simulink model "HVDCThyristorBased"  (R2024b)
settings: Solver=FixedStepDiscrete  StartTime=0.0  StopTime=2  FixedStep=Ts  RelTol=1e-3  AbsTol=1e-2
InitFcn:
  | Ts=50e-6;
  | 
  | % Rectifier AC side :
  | VLL_nom_R = 500e3; % V
  | Fnom_R = 60;           % Hz
  | 
  | % Inverter AC side :
  | VLL_nom_I = 345e3; % V
  | Fnom_I = 50;           % Hz
  | 
  | % DC :
  | Vdc_nom = 500e3;   % V
  | Idc_nom  = 2000;     % A
undefined symbols (not defined in the file or in its folder): D1, Delta, lagging, pulse, test_alpha
libraries: simulink x24, spsOnDelayLib x12, spsFirstOrderFilterLib x9, spsSampleandHoldLib x8, spsMultimeterLib x7, spsMonostableLib x7, spsThreePhaseHarmonicFilterLib x6, spsEdgeDetectorLib x6, spsGroundLib x4, spsUniversalBridgeLib x4, spsImpedanceMeasurementLib x3, spsBistableLib x3
(part 3 of 5)

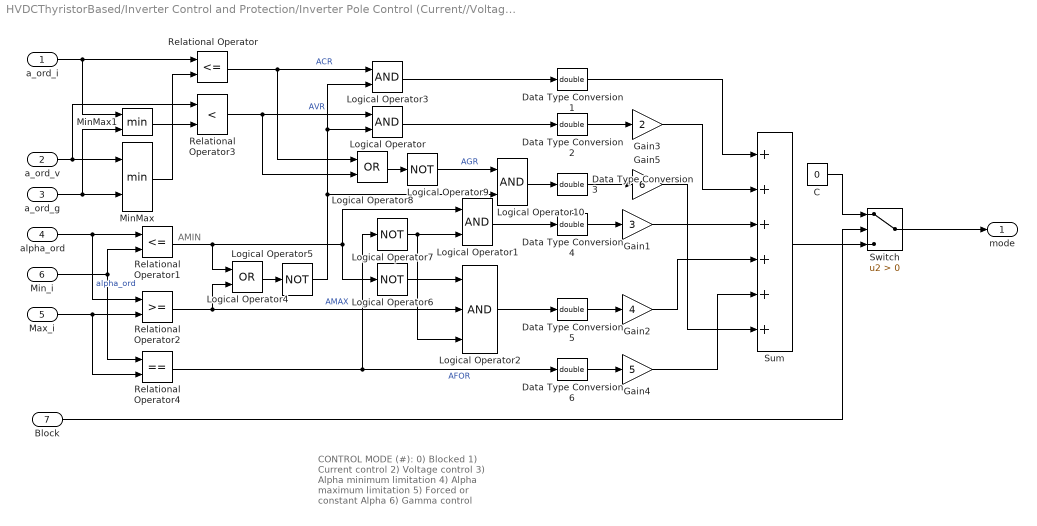
== system HVDCThyristorBased/Inverter Control and Protection/Inverter Pole Control (Current//Voltage//Gamma)/Control Mode  ==
  note: AMIN
  note: CONTROL MODE (#):
      |
      | 0) Blocked
      | 1) Current control
      | 2) Voltage control
      | 3) Alpha minimum limitation
      | 4) Alpha maximum limitation
      | 5) Forced or constant Alpha
      | 6) Gamma control
  "a_ord_i " : Inport
  a_ord_v : Inport  Port=2
  a_ord_g : Inport  Port=3
  alpha_ord : Inport  Port=4
  Max_i : Inport  Port=5
  Min_i : Inport  Port=6
  Block : Inport  Port=7
  C : Constant  Value=0
  Data Type Conversion{1..6} (6 alike) : DataTypeConversion  OutDataTypeStr=double  SaturateOnIntegerOverflow=off  RndMeth=Floor
  Gain1 : Gain  Gain=3  OutDataTypeStr=double  SaturateOnIntegerOverflow=on  ParamDataTypeStr=Inherit: Same as input
  Gain2 : Gain  Gain=4  OutDataTypeStr=double  SaturateOnIntegerOverflow=on  ParamDataTypeStr=Inherit: Same as input
  Gain3 : Gain  Gain=2  OutDataTypeStr=double  SaturateOnIntegerOverflow=on  ParamDataTypeStr=Inherit: Same as input
  Gain4 : Gain  Gain=5  OutDataTypeStr=double  SaturateOnIntegerOverflow=on  ParamDataTypeStr=Inherit: Same as input
  Gain5 : Gain  Gain=6  OutDataTypeStr=double  SaturateOnIntegerOverflow=on  ParamDataTypeStr=Inherit: Same as input
  Logical Operator{,1,3,10} (4 alike) : Logic
  Logical Operator2 : Logic  Inputs=3
  Logical Operator4 : Logic  Operator=OR
  Logical Operator{5..7,9} (4 alike) : Logic  Operator=NOT
  Logical Operator8 : Logic  Operator=OR
  MinMax : MinMax  Inputs=2  InputSameDT=on  SaturateOnIntegerOverflow=on
  MinMax1 : MinMax  Inputs=2  InputSameDT=on  SaturateOnIntegerOverflow=on
  Relational Operator : RelationalOperator  Operator=<=
  Relational Operator1 : RelationalOperator  Operator=<=
  Relational Operator2 : RelationalOperator
  Relational Operator3 : RelationalOperator  Operator=<
  Relational Operator4 : RelationalOperator  Operator===
  Sum : Sum  Inputs=++++++  InputSameDT=on  SaturateOnIntegerOverflow=on  OutDataTypeStr=Inherit: Same as first input
  Switch : Switch  Criteria=u2 > Threshold
  mode : Outport  VectorParamsAs1DForOutWhenUnconnected=off
  wires:
  Data Type Conversion6/1 -> Gain4/1
  Data Type Conversion5/1 -> Gain2/1
  Data Type Conversion4/1 -> Gain1/1
  Data Type Conversion3/1 -> Gain5/1
  Data Type Conversion2/1 -> Gain3/1
  Data Type Conversion1/1 -> Sum/1
  Switch/1 -> mode/1
  Logical Operator5/1 -> Logical Operator3/2, Logical Operator/2, Logical Operator10/2
  Logical Operator7/1 -> Logical Operator2/3, Logical Operator1/2
  Gain4/1 -> Sum/5
  Logical Operator1/1 -> Data Type Conversion4/1
  Relational Operator4/1 -> Logical Operator7/1, Data Type Conversion6/1  "AFOR"
  Max_i/1 -> Relational Operator4/2, Relational Operator2/2
  Min_i/1 -> Relational Operator4/1, Relational Operator1/2
  Gain2/1 -> Sum/4
  Gain1/1 -> Sum/3
  Logical Operator2/1 -> Data Type Conversion5/1
  Logical Operator6/1 -> Logical Operator2/1
  Relational Operator2/1 -> Logical Operator2/2, Logical Operator4/2  "AMAX"
  Logical Operator4/1 -> Logical Operator5/1
  Relational Operator1/1 -> Logical Operator1/1, Logical Operator6/1, Logical Operator4/1
  alpha_ord/1 -> Relational Operator2/1, Relational Operator1/1  "alpha_ord"
  Logical Operator/1 -> Data Type Conversion2/1
  Relational Operator3/1 -> Logical Operator/1, Logical Operator8/2  "AVR"
  Gain3/1 -> Sum/2
  Logical Operator3/1 -> Data Type Conversion1/1
  Relational Operator/1 -> Logical Operator3/1, Logical Operator8/1  "ACR"
  "a_ord_i "/1 -> Relational Operator/1, MinMax1/1
  Block/1 -> Switch/2
  Sum/1 -> Switch/3
  C/1 -> Switch/1
  a_ord_v/1 -> MinMax/1, Relational Operator3/1
  a_ord_g/1 -> MinMax/2, MinMax1/2
  MinMax/1 -> Relational Operator/2
  Logical Operator8/1 -> Logical Operator9/1
  Gain5/1 -> Sum/6
  MinMax1/1 -> Relational Operator3/2
  Logical Operator9/1 -> Logical Operator10/1  "AGR"
  Logical Operator10/1 -> Data Type Conversion3/1

== system HVDCThyristorBased/Inverter Control and Protection/Inverter Pole Control (Current//Voltage//Gamma)/Current Regulator ==
  note: Current Regulator
  Max_i : Inport
  Min_i : Inport  Port=2
  ERR : Inport  Port=3
  Max_pi : Inport  Port=4
  Min_pi : Inport  Port=5
  Alpha_lin : Inport  Port=6
  Max_lin : Inport  Port=7
  Min_lin : Inport  Port=8
  Inv : Inport  Port=9
  PI Regulator with external limits and linrarized Kp (Discrete) : Subsystem  mask(PI Regulator  With  External  Limits (Discrete)){Kp=Kp_I, Ki=Ki_I, IC_i=ICi_I, On_lin=on, pas=Ts}
      mask prompts: Kp "Kp (deg/pu):"; Ki "Ki (deg/pu/s):"; IC_i "Integrator Initial Condition (deg):"; On_lin "Linearization  (On)"; pas "Sample time (s):"
      mask help: For the linearization it is important to specifie the mode of operation i.e. rectifier or inverter (negation of rectifier).
      mask Display: disp('PI Regulator\nWith external limits\n(Linearized Kp)\n(Discrete)\n\n')
  Alpha_ord : Outport  VectorParamsAs1DForOutWhenUnconnected=off
  wires:
  PI Regulator with external limits and linrarized Kp (Discrete)/1(Alpha_ord) -> Alpha_ord/1
  Max_i/1 -> PI Regulator with external limits and linrarized Kp (Discrete)/1(Max_i)
  Min_i/1 -> PI Regulator with external limits and linrarized Kp (Discrete)/2(Min_i)
  ERR/1 -> PI Regulator with external limits and linrarized Kp (Discrete)/3(ERR)
  Max_pi/1 -> PI Regulator with external limits and linrarized Kp (Discrete)/4(Max_pi)
  Min_pi/1 -> PI Regulator with external limits and linrarized Kp (Discrete)/5(Min_pi)
  Alpha_lin/1 -> PI Regulator with external limits and linrarized Kp (Discrete)/6(Alpha_lin)
  Max_lin/1 -> PI Regulator with external limits and linrarized Kp (Discrete)/7(Max_lin)
  Min_lin/1 -> PI Regulator with external limits and linrarized Kp (Discrete)/8(Min_lin)
  Inv/1 -> PI Regulator with external limits and linrarized Kp (Discrete)/9(Inv)

== system HVDCThyristorBased/Inverter Control and Protection/Inverter Pole Control (Current//Voltage//Gamma)/Gamma Error ==
  note: Gamma Error
  G_ref : Inport
  G_meas : Inport  Port=2
  Block : Inport  Port=3
  Id_err : Inport  Port=4
  Enable (Held) : EnablePort  PropagateVarSize=During execution
  Constant1 : Constant  Value=0
  Constant2 : Constant  Value=0
  Constant3 : Constant  Value=G_marg
  Constant4 : Constant  Value=Id_marg
  First-Order Filter (T=0.01) : spsFirstOrderFilterLib/First-Order Filter  FilterType=Lowpass  Tc=0.01  Ts=Ts  Initialize=off  Vac_Init=[0, 0, 60]  Vdc_Init=0  PlotResponse=off  FreqRange="[0,  200,  1]"
  MIN:eps MAX:inf : Saturate  UpperLimit=inf  LowerLimit=eps
  Math Function : Math  Operator=reciprocal  SignedPower=on
  Product1 : Product  Inputs=3  InputSameDT=on  SaturateOnIntegerOverflow=on  OutDataTypeStr=Inherit: Same as first input
  Saturation Dynamic : simulink/Discontinuities/Saturation Dynamic  OutMin=[]  OutMax=[]  OutDataTypeStr=Inherit: Same as second input  OutDataType=fixdt(1, 16)  OutScaling=2^-10  DoSatur=off
  Sum3 : Sum  Inputs=-+-  InputSameDT=on  SaturateOnIntegerOverflow=on  OutDataTypeStr=Inherit: Same as first input
  Switch2 : Switch  Criteria=u2 > Threshold
  ERR_G : Outport  VectorParamsAs1DForOutWhenUnconnected=off
  wires:
  Saturation Dynamic/1 -> Product1/3
  Sum3/1 -> Switch2/3
  G_ref/1 -> Sum3/1
  G_meas/1 -> Sum3/2
  Constant1/1 -> Switch2/1
  Block/1 -> Switch2/2
  Switch2/1 -> ERR_G/1  "ERR"
  Constant2/1 -> Saturation Dynamic/3
  Math Function/1 -> Product1/2
  MIN:eps MAX:inf/1 -> Math Function/1
  Constant4/1 -> MIN:eps MAX:inf/1, Saturation Dynamic/1
  Product1/1 -> First-Order Filter (T=0.01)/1
  First-Order Filter (T=0.01)/1 -> Sum3/3  "dG"
  Id_err/1 -> Saturation Dynamic/2
  Constant3/1 -> Product1/1

== system HVDCThyristorBased/Inverter Control and Protection/Inverter Pole Control (Current//Voltage//Gamma)/Gamma Regulator ==
  note: Gamma Regulator
  Max_i : Inport
  Min_i : Inport  Port=2
  ERR : Inport  Port=3
  Max_pi : Inport  Port=4
  Min_pi : Inport  Port=5
  Alpha_lin : Inport  Port=6
  Max_lin : Inport  Port=7
  Min_lin : Inport  Port=8
  Inv : Inport  Port=9
  Enable (Held) : EnablePort  PropagateVarSize=During execution
  PI Regulator with external limits and linrarized Kp (Discrete)1 : Subsystem  mask(PI Regulator  With  External  Limits (Discrete)){Kp=Kp_G, Ki=Ki_G, IC_i=ICi_G, On_lin=on, pas=Ts}
      mask prompts: Kp "Kp (deg/pu):"; Ki "Ki (deg/pu/s):"; IC_i "Integrator Initial Condition (deg):"; On_lin "Linearization  (On)"; pas "Sample time (s):"
      mask help: For the linearization it is important to specifie the mode of operation i.e. rectifier or inverter (negation of rectifier).
      mask Display: disp('PI Regulator\nWith external limits\n(Linearized Kp)\n(Discrete)\n\n')
  Alpha_ord : Outport  VectorParamsAs1DForOutWhenUnconnected=off
  wires:
  PI Regulator with external limits and linrarized Kp (Discrete)1/1(Alpha_ord) -> Alpha_ord/1
  Max_i/1 -> PI Regulator with external limits and linrarized Kp (Discrete)1/1(Max_i)
  Min_i/1 -> PI Regulator with external limits and linrarized Kp (Discrete)1/2(Min_i)
  ERR/1 -> PI Regulator with external limits and linrarized Kp (Discrete)1/3(ERR)
  Max_pi/1 -> PI Regulator with external limits and linrarized Kp (Discrete)1/4(Max_pi)
  Min_pi/1 -> PI Regulator with external limits and linrarized Kp (Discrete)1/5(Min_pi)
  Alpha_lin/1 -> PI Regulator with external limits and linrarized Kp (Discrete)1/6(Alpha_lin)
  Max_lin/1 -> PI Regulator with external limits and linrarized Kp (Discrete)1/7(Max_lin)
  Min_lin/1 -> PI Regulator with external limits and linrarized Kp (Discrete)1/8(Min_lin)
  Inv/1 -> PI Regulator with external limits and linrarized Kp (Discrete)1/9(Inv)

== system HVDCThyristorBased/Inverter Control and Protection/Inverter Pole Control (Current//Voltage//Gamma)/Voltage Error ==
  note: Voltage Error
  Vd_ref : Inport
  Vd_meas : Inport  Port=2
  Block : Inport  Port=3
  Id_err : Inport  Port=4
  Enable (Held) : EnablePort  PropagateVarSize=During execution
  Constant1 : Constant  Value=0
  Constant2 : Constant  Value=0
  Constant3 : Constant  Value=Vd_marg
  Constant4 : Constant  Value=Id_marg
  First-Order Filter (T = 0.1) : spsFirstOrderFilterLib/First-Order Filter  FilterType=Lowpass  Tc=0.01  Ts=Ts  Initialize=on  Vac_Init=[0, 0, 60]  Vdc_Init=0  PlotResponse=off  FreqRange="[0,  200,  1]"
  MIN:eps MAX:inf : Saturate  UpperLimit=inf  LowerLimit=eps
  Math Function : Math  Operator=reciprocal  SignedPower=on
  Product1 : Product  Inputs=3  InputSameDT=on  SaturateOnIntegerOverflow=on  OutDataTypeStr=Inherit: Same as first input
  Saturation Dynamic : simulink/Discontinuities/Saturation Dynamic  OutMin=[]  OutMax=[]  OutDataTypeStr=Inherit: Same as second input  OutDataType=fixdt(1, 16)  OutScaling=2^-10  DoSatur=off
  Sum3 : Sum  Inputs=+--  InputSameDT=on  SaturateOnIntegerOverflow=on  OutDataTypeStr=Inherit: Same as first input
  Switch2 : Switch  Criteria=u2 > Threshold
  ERR_V : Outport  VectorParamsAs1DForOutWhenUnconnected=off
  wires:
  Saturation Dynamic/1 -> Product1/3
  Constant3/1 -> Product1/1
  Id_err/1 -> Saturation Dynamic/2
  First-Order Filter (T = 0.1)/1 -> Sum3/3  "dV"
  Product1/1 -> First-Order Filter (T = 0.1)/1
  Constant4/1 -> MIN:eps MAX:inf/1, Saturation Dynamic/1
  MIN:eps MAX:inf/1 -> Math Function/1
  Math Function/1 -> Product1/2
  Constant2/1 -> Saturation Dynamic/3
  Switch2/1 -> ERR_V/1  "ERR"
  Block/1 -> Switch2/2
  Constant1/1 -> Switch2/1
  Vd_meas/1 -> Sum3/2
  Vd_ref/1 -> Sum3/1
  Sum3/1 -> Switch2/3

== system HVDCThyristorBased/Inverter Control and Protection/Inverter Pole Control (Current//Voltage//Gamma)/Voltage Regulator ==
  note: Voltage Regulator
  Max_i : Inport
  Min_i : Inport  Port=2
  ERR : Inport  Port=3
  Max_pi : Inport  Port=4
  Min_pi : Inport  Port=5
  Alpha_lin : Inport  Port=6
  Max_lin : Inport  Port=7
  Min_lin : Inport  Port=8
  Inv : Inport  Port=9
  Enable (Held) : EnablePort  PropagateVarSize=During execution
  PI Regulator with external limits and linrarized Kp (Discrete) : Subsystem  mask(PI Regulator  With  External  Limits (Discrete)){Kp=Kp_V, Ki=Ki_V, IC_i=ICi_V, On_lin=on, pas=Ts}
      mask prompts: Kp "Kp (deg/pu):"; Ki "Ki (deg/pu/s):"; IC_i "Integrator Initial Condition (deg):"; On_lin "Linearization  (On)"; pas "Sample time (s):"
      mask help: For the linearization it is important to specifie the mode of operation i.e. rectifier or inverter (negation of rectifier).
      mask Display: disp('PI Regulator\nWith external limits\n(Linearized Kp)\n(Discrete)\n\n')
  Alpha_ord : Outport  VectorParamsAs1DForOutWhenUnconnected=off
  wires:
  Inv/1 -> PI Regulator with external limits and linrarized Kp (Discrete)/9(Inv)
  Min_lin/1 -> PI Regulator with external limits and linrarized Kp (Discrete)/8(Min_lin)
  Max_lin/1 -> PI Regulator with external limits and linrarized Kp (Discrete)/7(Max_lin)
  Alpha_lin/1 -> PI Regulator with external limits and linrarized Kp (Discrete)/6(Alpha_lin)
  Min_pi/1 -> PI Regulator with external limits and linrarized Kp (Discrete)/5(Min_pi)
  Max_pi/1 -> PI Regulator with external limits and linrarized Kp (Discrete)/4(Max_pi)
  ERR/1 -> PI Regulator with external limits and linrarized Kp (Discrete)/3(ERR)
  Min_i/1 -> PI Regulator with external limits and linrarized Kp (Discrete)/2(Min_i)
  Max_i/1 -> PI Regulator with external limits and linrarized Kp (Discrete)/1(Max_i)
  PI Regulator with external limits and linrarized Kp (Discrete)/1(Alpha_ord) -> Alpha_ord/1

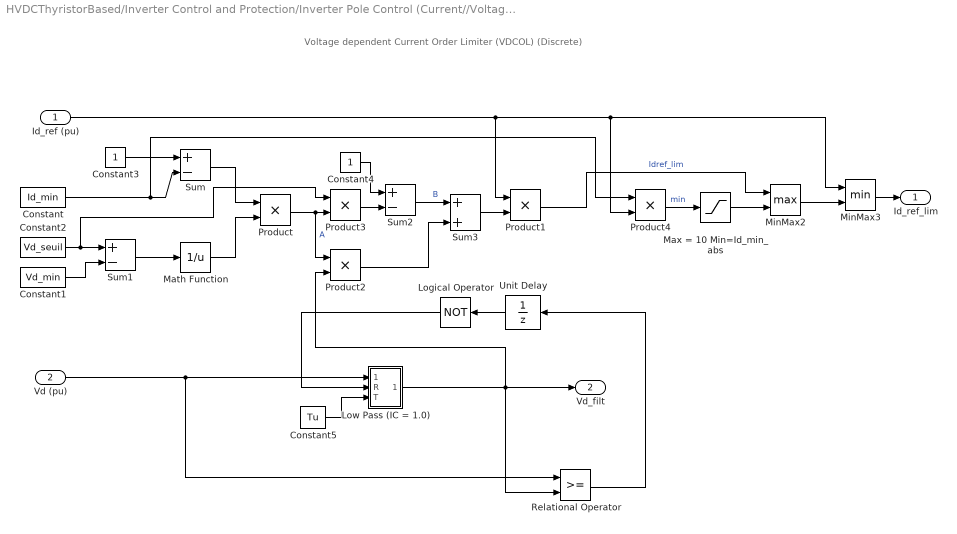
== system HVDCThyristorBased/Inverter Control and Protection/Inverter Pole Control (Current//Voltage//Gamma)/Voltage dependent Current Order Limiter ==
  note: Voltage dependent Current Order Limiter (VDCOL) (Discrete)
  Id_ref (pu) : Inport
  Vd (pu) : Inport  Port=2
  Constant : Constant  Value=Id_min
  Constant1 : Constant  Value=Vd_min
  Constant2 : Constant  Value=Vd_seuil
  Constant3 : Constant
  Constant4 : Constant
  Constant5 : Constant  Value=Tu
  Logical Operator : Logic  Operator=NOT
  Low Pass (IC = 1.0) : Subsystem  mask(Low Pass Filter With Reset (discrete: Zoh method, Forward Euler)){ic=1, dt=Ts}
      mask prompts: ic "Initial condition:"; dt "Sample time (s)"
      mask help:
      | The output will be reset to the input value (Time constant = 0)  during the input (2) is True. The Time constant (T) is defined by
      | input (3).
      mask Display:
      | plot(0,0,100,100,[90,80,70,60,50,40,29,20,10],[60,55,52,55,60,65,67,65,60],[89,80,71,60,50,40,30,20,10],[40,35,32,35,40,45,47,45,40],[56,44],[70,50]);
      | disp('\n\nD')
  Math Function : Math  Operator=reciprocal  SignedPower=on
  Max = 10 Min=Id_min_abs : Saturate  UpperLimit=10  LowerLimit=Id_min_abs
  MinMax2 : MinMax  Function=max  Inputs=2  InputSameDT=on  SaturateOnIntegerOverflow=on
  MinMax3 : MinMax  Inputs=2  InputSameDT=on  SaturateOnIntegerOverflow=on
  Product{,1..4} (5 alike) : Product  InputSameDT=on  SaturateOnIntegerOverflow=on  OutDataTypeStr=Inherit: Same as first input
  Relational Operator : RelationalOperator
  Sum : Sum  Inputs=+-  InputSameDT=on  SaturateOnIntegerOverflow=on  OutDataTypeStr=Inherit: Same as first input
  Sum1 : Sum  Inputs=+-  InputSameDT=on  SaturateOnIntegerOverflow=on  OutDataTypeStr=Inherit: Same as first input
  Sum2 : Sum  Inputs=+-  InputSameDT=on  SaturateOnIntegerOverflow=on  OutDataTypeStr=Inherit: Same as first input
  Sum3 : Sum  InputSameDT=on  SaturateOnIntegerOverflow=on  OutDataTypeStr=Inherit: Same as first input
  Unit Delay : UnitDelay  SampleTime=Ts  HasFrameUpgradeWarning=on
  Id_ref_lim : Outport  InitialOutput=0  VectorParamsAs1DForOutWhenUnconnected=off
  Vd_filt : Outport  Port=2  InitialOutput=0  VectorParamsAs1DForOutWhenUnconnected=off
  wires:
  Relational Operator/1 -> Unit Delay/1
  Max = 10 Min=Id_min_abs/1 -> MinMax2/2
  MinMax2/1 -> MinMax3/2
  Product1/1 -> MinMax2/1  "Idref_lim"
  Constant2/1 -> Product3/1, Sum1/1
  Product/1 -> Product3/2, Product2/1  "A"
  Product3/1 -> Sum2/2
  MinMax3/1 -> Id_ref_lim/1
  Id_ref (pu)/1 -> Product4/2, MinMax3/1, Product1/1
  Product4/1 -> Max = 10 Min=Id_min_abs/1  "min"
  Constant/1 -> Product4/1, Sum/2
  Sum3/1 -> Product1/2
  Product2/1 -> Sum3/2
  Sum2/1 -> Sum3/1  "B"
  Constant4/1 -> Sum2/1
  Math Function/1 -> Product/2
  Sum/1 -> Product/1
  Sum1/1 -> Math Function/1
  Constant1/1 -> Sum1/2
  Constant3/1 -> Sum/1
  Constant5/1 -> Low Pass (IC = 1.0)/3(T)
  Low Pass (IC = 1.0)/1(Out) -> Vd_filt/1, Relational Operator/2, Product2/2
  Vd (pu)/1 -> Relational Operator/1, Low Pass (IC = 1.0)/1(In)
  Unit Delay/1 -> Logical Operator/1
  Logical Operator/1 -> Low Pass (IC = 1.0)/2(R)

== system HVDCThyristorBased/Inverter Control and Protection/Inverter Pole Control (Current//Voltage//Gamma)/alpha_init ==
  In1 : Inport  PortDimensions=1
  IC : InitialCondition  Value=min([ICi_V,ICi_I,ICi_G])
  Out1 : Outport  VectorParamsAs1DForOutWhenUnconnected=off
  wires:
  IC/1 -> Out1/1
  In1/1 -> IC/1

== system HVDCThyristorBased/Inverter Control and Protection/Inverter Protections/Commutation Failure Prevention Control (CFPREV) ==
  note: Commutation failure Prevention Control Module (CFPREV)
  Uabc (pu) : Inport
  C : Constant  Value=STATE
  CFPREV : Subsystem  TreatAsAtomicUnit=on
  AMIN_CFPREV (deg) : Outport  VectorParamsAs1DForOutWhenUnconnected=off
  wires:
  C/1 -> CFPREV/Enable
  Uabc (pu)/1 -> CFPREV/1(Uabc (pu))
  CFPREV/1(AMIN_CFPREV (deg)) -> AMIN_CFPREV (deg)/1

== system HVDCThyristorBased/Inverter Control and Protection/Inverter Protections/Informations ==
  note: The CFPREV  mitigates commutation failures due to AC voltage dips. After a fault detection (three-phase or
      | one-phase) an angle value (AMIN_CFPREV) is sent to the converter control in order to be deducted from the
      | maximum delay angle limit (alpha_max). In practice, the commutation margin is consequently enlarged
      | reducing therefore the risk of commutation failures (note 1).
  note: The Commutation failure prevention control (CFPREV) and the Low AC voltage detection (LACVD)
      | constitutes the protective functions at the rinverter.
  note: The LACVD detects a low AC voltage condition on the inverter commutation bus and sends a signal
      | (Lock) to the DCPROT (in the rectifier) in order to prevent the detection of a DC fault when the drop in
      | the DC voltage is due to a fault on the AC side. The LACVD at the irectifier sends also a signal to
      | lock the DCPROT for the same reason.
  note: DESCRIPTION
  note: DC Protections - Inverter
  note: NOTE 1: Result of a failure of the incoming valve to take over the direct current before the commutating voltage reverses its polarity.

== system HVDCThyristorBased/Inverter Control and Protection/Inverter Protections/Low  AC Voltage Detection (LACVD) ==
  note: Low AC Voltage Detection
  Uac (pu) : Inport
  Enable (Held) : EnablePort  PropagateVarSize=During execution  ShowOutputPort=on
  C : Constant  Value=STATE
  LACVD : Subsystem  TreatAsAtomicUnit=on
  Logical Operator : Logic  AllPortsSameDT=off
  Low_AC_Voltage : Outport  VectorParamsAs1DForOutWhenUnconnected=off
  wires:
  Uac (pu)/1 -> LACVD/1(Uac (pu))
  LACVD/1(Low_AC_Voltage) -> Low_AC_Voltage/1
  Enable (Held)/1 -> Logical Operator/1
  Logical Operator/1 -> LACVD/Enable
  C/1 -> Logical Operator/2

== system HVDCThyristorBased/Inverter Control and Protection/Inverter Protections/Udio_6p ==
  note: Three-phase full-wave rectification
  Uabc (pu) : Inport
  MinMax : MinMax  Function=max  InputSameDT=on  SaturateOnIntegerOverflow=on
  MinMax1 : MinMax  InputSameDT=on  SaturateOnIntegerOverflow=on
  Sum : Sum  Inputs=+-  InputSameDT=on  SaturateOnIntegerOverflow=on  OutDataTypeStr=Inherit: Same as first input
  conversion pu ac->dc : Gain  Gain=pi/(3*sqrt(3))  SaturateOnIntegerOverflow=on  OutDataTypeStr=Inherit: Same as input  ParamDataTypeStr=Inherit: Same as input
  Udio_6p : Outport  VectorParamsAs1DForOutWhenUnconnected=off
  wires:
  conversion pu ac->dc/1 -> Udio_6p/1
  Sum/1 -> conversion pu ac->dc/1
  Uabc (pu)/1 -> MinMax1/1, MinMax/1
  MinMax/1 -> Sum/1
  MinMax1/1 -> Sum/2

== system HVDCThyristorBased/Master Control/Start//Stop/S1 ==
  Start : Inport
  Down : Constant  Value=0
  Ramp : FromWorkspace  VariableName="[T_ramp,  U_ramp]"  SampleTime=Ts  ZeroCross=off
  Start-Stop Ramp : RateLimiter  RisingSlewLimit=SS_ramp  FallingSlewLimit=-SS_ramp
  Sum : Sum  InputSameDT=on  SaturateOnIntegerOverflow=on  OutDataTypeStr=Inherit: Same as first input
  Switch : Switch  Criteria=u2 > Threshold  InputSameDT=off
  UP : Constant  Value=Min_ref
  Out1 : Outport  InitialOutput=0  VectorParamsAs1DForOutWhenUnconnected=off
  wires:
  Sum/1 -> Out1/1
  Ramp/1 -> Sum/1
  Start/1 -> Switch/2
  Switch/1 -> Start-Stop Ramp/1
  Down/1 -> Switch/3
  UP/1 -> Switch/1
  Start-Stop Ramp/1 -> Sum/2

== system HVDCThyristorBased/Rectifier Control and Protection/Rectifier Pole Control (Current)/Alpha Control ==
  note: Alpha Control
  Forced_alpha : Inport
  D_alpha : Inport  Port=2
  Constant1 : Constant  Value=alpha_min
  Constant2 : Constant  Value=alpha_max
  Constant3 : Constant  Value=test_alpha
  Data Type Conversion : DataTypeConversion  OutDataTypeStr=boolean
  Logical Operator : Logic  Operator=OR
  "Rate Limiter (Rate limit) " : RateLimiter  RisingSlewLimit=PRate_fix  FallingSlewLimit=NRate_fix
  "Rate Limiter (Rate limit)    " : RateLimiter  RisingSlewLimit=PRate_fix  FallingSlewLimit=NRate_fix
  Sum : Sum  Inputs=-+  InputSameDT=on  SaturateOnIntegerOverflow=on  OutDataTypeStr=Inherit: Same as first input
  Switch : Switch  Criteria=u2 > Threshold
  Switch1 : Switch  Criteria=u2 > Threshold
  fixed alpha (deg) : Constant  Value=alpha_fix
  Max_i : Outport  VectorParamsAs1DForOutWhenUnconnected=off
  Min_i : Outport  Port=2  VectorParamsAs1DForOutWhenUnconnected=off
  wires:
  "Rate Limiter (Rate limit)    "/1 -> Min_i/1
  "Rate Limiter (Rate limit) "/1 -> Max_i/1
  D_alpha/1 -> Sum/1
  Sum/1 -> Switch/3
  Constant2/1 -> Sum/2
  Constant3/1 -> Logical Operator/1
  Logical Operator/1 -> Switch/2, Switch1/2
  Constant1/1 -> Switch1/3
  Switch/1 -> "Rate Limiter (Rate limit) "/1
  Switch1/1 -> "Rate Limiter (Rate limit)    "/1
  fixed alpha (deg)/1 -> Switch/1, Switch1/1
  Forced_alpha/1 -> Data Type Conversion/1
  Data Type Conversion/1 -> Logical Operator/2

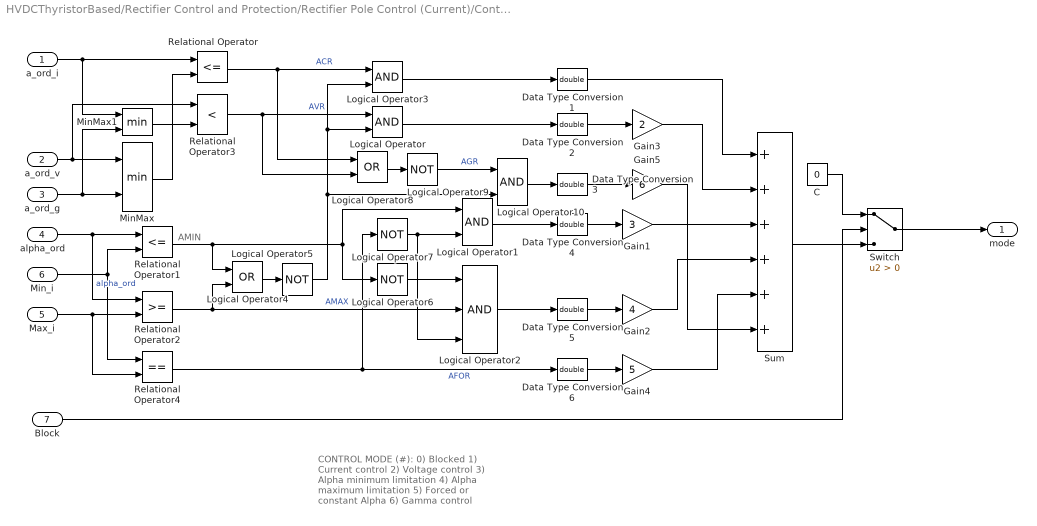
== system HVDCThyristorBased/Rectifier Control and Protection/Rectifier Pole Control (Current)/Control Mode  ==
  note: AMIN
  note: CONTROL MODE (#):
      |
      | 0) Blocked
      | 1) Current control
      | 2) Voltage control
      | 3) Alpha minimum limitation
      | 4) Alpha maximum limitation
      | 5) Forced or constant Alpha
      | 6) Gamma control
  "a_ord_i " : Inport
  a_ord_v : Inport  Port=2
  a_ord_g : Inport  Port=3
  alpha_ord : Inport  Port=4
  Max_i : Inport  Port=5
  Min_i : Inport  Port=6
  Block : Inport  Port=7
  C : Constant  Value=0
  Data Type Conversion{1..6} (6 alike) : DataTypeConversion  OutDataTypeStr=double  SaturateOnIntegerOverflow=off  RndMeth=Floor
  Gain1 : Gain  Gain=3  OutDataTypeStr=double  SaturateOnIntegerOverflow=on  ParamDataTypeStr=Inherit: Same as input
  Gain2 : Gain  Gain=4  OutDataTypeStr=double  SaturateOnIntegerOverflow=on  ParamDataTypeStr=Inherit: Same as input
  Gain3 : Gain  Gain=2  OutDataTypeStr=double  SaturateOnIntegerOverflow=on  ParamDataTypeStr=Inherit: Same as input
  Gain4 : Gain  Gain=5  OutDataTypeStr=double  SaturateOnIntegerOverflow=on  ParamDataTypeStr=Inherit: Same as input
  Gain5 : Gain  Gain=6  OutDataTypeStr=double  SaturateOnIntegerOverflow=on  ParamDataTypeStr=Inherit: Same as input
  Logical Operator{,1,3,10} (4 alike) : Logic
  Logical Operator2 : Logic  Inputs=3
  Logical Operator4 : Logic  Operator=OR
  Logical Operator{5..7,9} (4 alike) : Logic  Operator=NOT
  Logical Operator8 : Logic  Operator=OR
  MinMax : MinMax  Inputs=2  InputSameDT=on  SaturateOnIntegerOverflow=on
  MinMax1 : MinMax  Inputs=2  InputSameDT=on  SaturateOnIntegerOverflow=on
  Relational Operator : RelationalOperator  Operator=<=
  Relational Operator1 : RelationalOperator  Operator=<=
  Relational Operator2 : RelationalOperator
  Relational Operator3 : RelationalOperator  Operator=<
  Relational Operator4 : RelationalOperator  Operator===
  Sum : Sum  Inputs=++++++  InputSameDT=on  SaturateOnIntegerOverflow=on  OutDataTypeStr=Inherit: Same as first input
  Switch : Switch  Criteria=u2 > Threshold
  mode : Outport  VectorParamsAs1DForOutWhenUnconnected=off
  wires:
  Data Type Conversion6/1 -> Gain4/1
  Data Type Conversion5/1 -> Gain2/1
  Data Type Conversion4/1 -> Gain1/1
  Data Type Conversion3/1 -> Gain5/1
  Data Type Conversion2/1 -> Gain3/1
  Data Type Conversion1/1 -> Sum/1
  Switch/1 -> mode/1
  Logical Operator5/1 -> Logical Operator3/2, Logical Operator/2, Logical Operator10/2
  Logical Operator7/1 -> Logical Operator2/3, Logical Operator1/2
  Gain4/1 -> Sum/5
  Logical Operator1/1 -> Data Type Conversion4/1
  Relational Operator4/1 -> Logical Operator7/1, Data Type Conversion6/1  "AFOR"
  Max_i/1 -> Relational Operator4/2, Relational Operator2/2
  Min_i/1 -> Relational Operator4/1, Relational Operator1/2
  Gain2/1 -> Sum/4
  Gain1/1 -> Sum/3
  Logical Operator2/1 -> Data Type Conversion5/1
  Logical Operator6/1 -> Logical Operator2/1
  Relational Operator2/1 -> Logical Operator2/2, Logical Operator4/2  "AMAX"
  Logical Operator4/1 -> Logical Operator5/1
  Relational Operator1/1 -> Logical Operator1/1, Logical Operator6/1, Logical Operator4/1
  alpha_ord/1 -> Relational Operator2/1, Relational Operator1/1  "alpha_ord"
  Logical Operator/1 -> Data Type Conversion2/1
  Relational Operator3/1 -> Logical Operator/1, Logical Operator8/2  "AVR"
  Gain3/1 -> Sum/2
  Logical Operator3/1 -> Data Type Conversion1/1
  Relational Operator/1 -> Logical Operator3/1, Logical Operator8/1  "ACR"
  "a_ord_i "/1 -> Relational Operator/1, MinMax1/1
  Block/1 -> Switch/2
  Sum/1 -> Switch/3
  C/1 -> Switch/1
  a_ord_v/1 -> MinMax/1, Relational Operator3/1
  a_ord_g/1 -> MinMax/2, MinMax1/2
  MinMax/1 -> Relational Operator/2
  Logical Operator8/1 -> Logical Operator9/1
  Gain5/1 -> Sum/6
  MinMax1/1 -> Relational Operator3/2
  Logical Operator9/1 -> Logical Operator10/1  "AGR"
  Logical Operator10/1 -> Data Type Conversion3/1

== system HVDCThyristorBased/Rectifier Control and Protection/Rectifier Pole Control (Current)/Current Regulator ==
  note: Current Regulator
  Max_i : Inport
  Min_i : Inport  Port=2
  ERR : Inport  Port=3
  Max_pi : Inport  Port=4
  Min_pi : Inport  Port=5
  Alpha_lin : Inport  Port=6
  Max_lin : Inport  Port=7
  Min_lin : Inport  Port=8
  Inv : Inport  Port=9
  PI Regulator with external limits and linrarized Kp (Discrete) : Subsystem  mask(PI Regulator  With  External  Limits (Discrete)){Kp=Kp_I, Ki=Ki_I, IC_i=ICi_I, On_lin=on, pas=Ts}
      mask prompts: Kp "Kp (deg/pu):"; Ki "Ki (deg/pu/s):"; IC_i "Integrator Initial Condition (deg):"; On_lin "Linearization  (On)"; pas "Sample time (s):"
      mask help: For the linearization it is important to specifie the mode of operation i.e. rectifier or inverter (negation of rectifier).
      mask Display: disp('PI Regulator\nWith external limits\n(Linearized Kp)\n(Discrete)\n\n')
  Alpha_ord : Outport  VectorParamsAs1DForOutWhenUnconnected=off
  wires:
  PI Regulator with external limits and linrarized Kp (Discrete)/1(Alpha_ord) -> Alpha_ord/1
  Max_i/1 -> PI Regulator with external limits and linrarized Kp (Discrete)/1(Max_i)
  Min_i/1 -> PI Regulator with external limits and linrarized Kp (Discrete)/2(Min_i)
  ERR/1 -> PI Regulator with external limits and linrarized Kp (Discrete)/3(ERR)
  Max_pi/1 -> PI Regulator with external limits and linrarized Kp (Discrete)/4(Max_pi)
  Min_pi/1 -> PI Regulator with external limits and linrarized Kp (Discrete)/5(Min_pi)
  Alpha_lin/1 -> PI Regulator with external limits and linrarized Kp (Discrete)/6(Alpha_lin)
  Max_lin/1 -> PI Regulator with external limits and linrarized Kp (Discrete)/7(Max_lin)
  Min_lin/1 -> PI Regulator with external limits and linrarized Kp (Discrete)/8(Min_lin)
  Inv/1 -> PI Regulator with external limits and linrarized Kp (Discrete)/9(Inv)

== system HVDCThyristorBased/Rectifier Control and Protection/Rectifier Pole Control (Current)/Gamma Error ==
  note: Gamma Error
  G_ref : Inport
  G_meas : Inport  Port=2
  Block : Inport  Port=3
  Id_err : Inport  Port=4
  Enable (Held) : EnablePort  PropagateVarSize=During execution
  Constant1 : Constant  Value=0
  Constant2 : Constant  Value=0
  Constant3 : Constant  Value=G_marg
  Constant4 : Constant  Value=Id_marg
  First-Order Filter (T=0.01) : spsFirstOrderFilterLib/First-Order Filter  FilterType=Lowpass  Tc=0.01  Ts=Ts  Initialize=off  Vac_Init=[0, 0, 60]  Vdc_Init=0  PlotResponse=off  FreqRange="[0,  200,  1]"
  MIN:eps MAX:inf : Saturate  UpperLimit=inf  LowerLimit=eps
  Math Function : Math  Operator=reciprocal  SignedPower=on
  Product1 : Product  Inputs=3  InputSameDT=on  SaturateOnIntegerOverflow=on  OutDataTypeStr=Inherit: Same as first input
  Saturation Dynamic : simulink/Discontinuities/Saturation Dynamic  OutMin=[]  OutMax=[]  OutDataTypeStr=Inherit: Same as second input  OutDataType=fixdt(1, 16)  OutScaling=2^-10  DoSatur=off
  Sum3 : Sum  Inputs=-+-  InputSameDT=on  SaturateOnIntegerOverflow=on  OutDataTypeStr=Inherit: Same as first input
  Switch2 : Switch  Criteria=u2 > Threshold
  ERR_G : Outport  VectorParamsAs1DForOutWhenUnconnected=off
  wires:
  Saturation Dynamic/1 -> Product1/3
  Sum3/1 -> Switch2/3
  G_ref/1 -> Sum3/1
  G_meas/1 -> Sum3/2
  Constant1/1 -> Switch2/1
  Block/1 -> Switch2/2
  Switch2/1 -> ERR_G/1  "ERR"
  Constant2/1 -> Saturation Dynamic/3
  Math Function/1 -> Product1/2
  MIN:eps MAX:inf/1 -> Math Function/1
  Constant4/1 -> MIN:eps MAX:inf/1, Saturation Dynamic/1
  Product1/1 -> First-Order Filter (T=0.01)/1
  First-Order Filter (T=0.01)/1 -> Sum3/3  "dG"
  Id_err/1 -> Saturation Dynamic/2
  Constant3/1 -> Product1/1

== system HVDCThyristorBased/Rectifier Control and Protection/Rectifier Pole Control (Current)/Gamma Regulator ==
  note: Gamma Regulator
  Max_i : Inport
  Min_i : Inport  Port=2
  ERR : Inport  Port=3
  Max_pi : Inport  Port=4
  Min_pi : Inport  Port=5
  Alpha_lin : Inport  Port=6
  Max_lin : Inport  Port=7
  Min_lin : Inport  Port=8
  Inv : Inport  Port=9
  Enable (Held) : EnablePort  PropagateVarSize=During execution
  PI Regulator with external limits and linrarized Kp (Discrete)1 : Subsystem  mask(PI Regulator  With  External  Limits (Discrete)){Kp=Kp_G, Ki=Ki_G, IC_i=ICi_G, On_lin=on, pas=Ts}
      mask prompts: Kp "Kp (deg/pu):"; Ki "Ki (deg/pu/s):"; IC_i "Integrator Initial Condition (deg):"; On_lin "Linearization  (On)"; pas "Sample time (s):"
      mask help: For the linearization it is important to specifie the mode of operation i.e. rectifier or inverter (negation of rectifier).
      mask Display: disp('PI Regulator\nWith external limits\n(Linearized Kp)\n(Discrete)\n\n')
  Alpha_ord : Outport  VectorParamsAs1DForOutWhenUnconnected=off
  wires:
  PI Regulator with external limits and linrarized Kp (Discrete)1/1(Alpha_ord) -> Alpha_ord/1
  Max_i/1 -> PI Regulator with external limits and linrarized Kp (Discrete)1/1(Max_i)
  Min_i/1 -> PI Regulator with external limits and linrarized Kp (Discrete)1/2(Min_i)
  ERR/1 -> PI Regulator with external limits and linrarized Kp (Discrete)1/3(ERR)
  Max_pi/1 -> PI Regulator with external limits and linrarized Kp (Discrete)1/4(Max_pi)
  Min_pi/1 -> PI Regulator with external limits and linrarized Kp (Discrete)1/5(Min_pi)
  Alpha_lin/1 -> PI Regulator with external limits and linrarized Kp (Discrete)1/6(Alpha_lin)
  Max_lin/1 -> PI Regulator with external limits and linrarized Kp (Discrete)1/7(Max_lin)
  Min_lin/1 -> PI Regulator with external limits and linrarized Kp (Discrete)1/8(Min_lin)
  Inv/1 -> PI Regulator with external limits and linrarized Kp (Discrete)1/9(Inv)

== system HVDCThyristorBased/Rectifier Control and Protection/Rectifier Pole Control (Current)/Voltage Error ==
  note: Voltage Error
  Vd_ref : Inport
  Vd_meas : Inport  Port=2
  Block : Inport  Port=3
  Id_err : Inport  Port=4
  Enable (Held) : EnablePort  PropagateVarSize=During execution
  Constant1 : Constant  Value=0
  Constant2 : Constant  Value=0
  Constant3 : Constant  Value=Vd_marg
  Constant4 : Constant  Value=Id_marg
  First-Order Filter (T = 0.1) : spsFirstOrderFilterLib/First-Order Filter  FilterType=Lowpass  Tc=0.01  Ts=Ts  Initialize=on  Vac_Init=[0, 0, 60]  Vdc_Init=0  PlotResponse=off  FreqRange="[0,  200,  1]"
  MIN:eps MAX:inf : Saturate  UpperLimit=inf  LowerLimit=eps
  Math Function : Math  Operator=reciprocal  SignedPower=on
  Product1 : Product  Inputs=3  InputSameDT=on  SaturateOnIntegerOverflow=on  OutDataTypeStr=Inherit: Same as first input
  Saturation Dynamic : simulink/Discontinuities/Saturation Dynamic  OutMin=[]  OutMax=[]  OutDataTypeStr=Inherit: Same as second input  OutDataType=fixdt(1, 16)  OutScaling=2^-10  DoSatur=off
  Sum3 : Sum  Inputs=+--  InputSameDT=on  SaturateOnIntegerOverflow=on  OutDataTypeStr=Inherit: Same as first input
  Switch2 : Switch  Criteria=u2 > Threshold
  ERR_V : Outport  VectorParamsAs1DForOutWhenUnconnected=off
  wires:
  Saturation Dynamic/1 -> Product1/3
  Constant3/1 -> Product1/1
  Id_err/1 -> Saturation Dynamic/2
  First-Order Filter (T = 0.1)/1 -> Sum3/3  "dV"
  Product1/1 -> First-Order Filter (T = 0.1)/1
  Constant4/1 -> MIN:eps MAX:inf/1, Saturation Dynamic/1
  MIN:eps MAX:inf/1 -> Math Function/1
  Math Function/1 -> Product1/2
  Constant2/1 -> Saturation Dynamic/3
  Switch2/1 -> ERR_V/1  "ERR"
  Block/1 -> Switch2/2
  Constant1/1 -> Switch2/1
  Vd_meas/1 -> Sum3/2
  Vd_ref/1 -> Sum3/1
  Sum3/1 -> Switch2/3

== system HVDCThyristorBased/Rectifier Control and Protection/Rectifier Pole Control (Current)/Voltage Regulator ==
  note: Voltage Regulator
  Max_i : Inport
  Min_i : Inport  Port=2
  ERR : Inport  Port=3
  Max_pi : Inport  Port=4
  Min_pi : Inport  Port=5
  Alpha_lin : Inport  Port=6
  Max_lin : Inport  Port=7
  Min_lin : Inport  Port=8
  Inv : Inport  Port=9
  Enable (Held) : EnablePort  PropagateVarSize=During execution
  PI Regulator with external limits and linrarized Kp (Discrete) : Subsystem  mask(PI Regulator  With  External  Limits (Discrete)){Kp=Kp_V, Ki=Ki_V, IC_i=ICi_V, On_lin=on, pas=Ts}
      mask prompts: Kp "Kp (deg/pu):"; Ki "Ki (deg/pu/s):"; IC_i "Integrator Initial Condition (deg):"; On_lin "Linearization  (On)"; pas "Sample time (s):"
      mask help: For the linearization it is important to specifie the mode of operation i.e. rectifier or inverter (negation of rectifier).
      mask Display: disp('PI Regulator\nWith external limits\n(Linearized Kp)\n(Discrete)\n\n')
  Alpha_ord : Outport  VectorParamsAs1DForOutWhenUnconnected=off
  wires:
  Inv/1 -> PI Regulator with external limits and linrarized Kp (Discrete)/9(Inv)
  Min_lin/1 -> PI Regulator with external limits and linrarized Kp (Discrete)/8(Min_lin)
  Max_lin/1 -> PI Regulator with external limits and linrarized Kp (Discrete)/7(Max_lin)
  Alpha_lin/1 -> PI Regulator with external limits and linrarized Kp (Discrete)/6(Alpha_lin)
  Min_pi/1 -> PI Regulator with external limits and linrarized Kp (Discrete)/5(Min_pi)
  Max_pi/1 -> PI Regulator with external limits and linrarized Kp (Discrete)/4(Max_pi)
  ERR/1 -> PI Regulator with external limits and linrarized Kp (Discrete)/3(ERR)
  Min_i/1 -> PI Regulator with external limits and linrarized Kp (Discrete)/2(Min_i)
  Max_i/1 -> PI Regulator with external limits and linrarized Kp (Discrete)/1(Max_i)
  PI Regulator with external limits and linrarized Kp (Discrete)/1(Alpha_ord) -> Alpha_ord/1

== system HVDCThyristorBased/Rectifier Control and Protection/Rectifier Pole Control (Current)/Voltage dependent Current Order Limiter ==
  note: Voltage dependent Current Order Limiter (VDCOL) (Discrete)
  Id_ref (pu) : Inport
  Vd (pu) : Inport  Port=2
  Constant : Constant  Value=Id_min
  Constant1 : Constant  Value=Vd_min
  Constant2 : Constant  Value=Vd_seuil
  Constant3 : Constant
  Constant4 : Constant
  Constant5 : Constant  Value=Tu
  Logical Operator : Logic  Operator=NOT
  Low Pass (IC = 1.0) : Subsystem  mask(Low Pass Filter With Reset (discrete: Zoh method, Forward Euler)){ic=1, dt=Ts}
      mask prompts: ic "Initial condition:"; dt "Sample time (s)"
      mask help:
      | The output will be reset to the input value (Time constant = 0)  during the input (2) is True. The Time constant (T) is defined by
      | input (3).
      mask Display:
      | plot(0,0,100,100,[90,80,70,60,50,40,29,20,10],[60,55,52,55,60,65,67,65,60],[89,80,71,60,50,40,30,20,10],[40,35,32,35,40,45,47,45,40],[56,44],[70,50]);
      | disp('\n\nD')
  Math Function : Math  Operator=reciprocal  SignedPower=on
  Max = 10 Min=Id_min_abs : Saturate  UpperLimit=10  LowerLimit=Id_min_abs
  MinMax2 : MinMax  Function=max  Inputs=2  InputSameDT=on  SaturateOnIntegerOverflow=on
  MinMax3 : MinMax  Inputs=2  InputSameDT=on  SaturateOnIntegerOverflow=on
  Product{,1..4} (5 alike) : Product  InputSameDT=on  SaturateOnIntegerOverflow=on  OutDataTypeStr=Inherit: Same as first input
  Relational Operator : RelationalOperator
  Sum : Sum  Inputs=+-  InputSameDT=on  SaturateOnIntegerOverflow=on  OutDataTypeStr=Inherit: Same as first input
  Sum1 : Sum  Inputs=+-  InputSameDT=on  SaturateOnIntegerOverflow=on  OutDataTypeStr=Inherit: Same as first input
  Sum2 : Sum  Inputs=+-  InputSameDT=on  SaturateOnIntegerOverflow=on  OutDataTypeStr=Inherit: Same as first input
  Sum3 : Sum  InputSameDT=on  SaturateOnIntegerOverflow=on  OutDataTypeStr=Inherit: Same as first input
  Unit Delay : UnitDelay  SampleTime=Ts  HasFrameUpgradeWarning=on
  Id_ref_lim : Outport  InitialOutput=0  VectorParamsAs1DForOutWhenUnconnected=off
  Vd_filt : Outport  Port=2  InitialOutput=0  VectorParamsAs1DForOutWhenUnconnected=off
  wires:
  Relational Operator/1 -> Unit Delay/1
  Max = 10 Min=Id_min_abs/1 -> MinMax2/2
  MinMax2/1 -> MinMax3/2
  Product1/1 -> MinMax2/1  "Idref_lim"
  Constant2/1 -> Product3/1, Sum1/1
  Product/1 -> Product3/2, Product2/1  "A"
  Product3/1 -> Sum2/2
  MinMax3/1 -> Id_ref_lim/1
  Id_ref (pu)/1 -> Product4/2, MinMax3/1, Product1/1
  Product4/1 -> Max = 10 Min=Id_min_abs/1  "min"
  Constant/1 -> Product4/1, Sum/2
  Sum3/1 -> Product1/2
  Product2/1 -> Sum3/2
  Sum2/1 -> Sum3/1  "B"
  Constant4/1 -> Sum2/1
  Math Function/1 -> Product/2
  Sum/1 -> Product/1
  Sum1/1 -> Math Function/1
  Constant1/1 -> Sum1/2
  Constant3/1 -> Sum/1
  Constant5/1 -> Low Pass (IC = 1.0)/3(T)
  Low Pass (IC = 1.0)/1(Out) -> Vd_filt/1, Relational Operator/2, Product2/2
  Vd (pu)/1 -> Relational Operator/1, Low Pass (IC = 1.0)/1(In)
  Unit Delay/1 -> Logical Operator/1
  Logical Operator/1 -> Low Pass (IC = 1.0)/2(R)

== system HVDCThyristorBased/Rectifier Control and Protection/Rectifier Pole Control (Current)/alpha_init ==
  In1 : Inport  PortDimensions=1
  IC : InitialCondition  Value=min([ICi_V,ICi_I,ICi_G])
  Out1 : Outport  VectorParamsAs1DForOutWhenUnconnected=off
  wires:
  IC/1 -> Out1/1
  In1/1 -> IC/1

== system HVDCThyristorBased/Rectifier Control and Protection/Rectifier Protections/DC Fault Protection (DCPROT) ==
  note: DC Fault Protection (only in Rectifier)
  VdL (pu) : Inport
  Deblocked : Inport  Port=2  OutDataTypeStr=boolean
  Lock : Inport  Port=3
  (Held) : EnablePort  PropagateVarSize=During execution  ShowOutputPort=on
  C : Constant  Value=STATE
  Enabled Subsystem : Subsystem  TreatAsAtomicUnit=on
  Logical Operator : Logic  AllPortsSameDT=off
  Forced_alpha : Outport  VectorParamsAs1DForOutWhenUnconnected=off
  wires:
  (Held)/1 -> Logical Operator/1
  C/1 -> Logical Operator/2
  Logical Operator/1 -> Enabled Subsystem/Enable
  VdL (pu)/1 -> Enabled Subsystem/1(VdL (pu))
  Lock/1 -> Enabled Subsystem/3(Lock)
  Deblocked/1 -> Enabled Subsystem/2(Deblocked)
  Enabled Subsystem/1(Forced_alpha) -> Forced_alpha/1

== system HVDCThyristorBased/Rectifier Control and Protection/Rectifier Protections/Informations ==
  note: The  DCPROT detects a fault on the DC line and tries to extinguish the fault current by ordering a Forced
      | alpha operation for a fixed duration.
  note: The LACVD detects a low AC voltage condition on the rectifier commutation bus and sends a signal
      | (Lock) to the DCPROT in order to prevent the detection of a DC fault when the drop in the DC voltage is
      | due to a fault on the AC side. The LACVD at the inverter sends also a signal to lock the DCPROT for the
      | same reason.
  note: DC Protections - Rectifier
  note: Silvano Casoria (Hydro-Quebec)
  note: DESCRIPTION
  note: The DC fault protection (DCPROT) and the Low AC voltage detection (LACVD) constitutes the
      | protectives functions at the rectifier. The DC fault protection detects a fault on the DC line and tries to
      | extinguish the fault current by ordering a Forced alpha operation during a fixed duration.

== system HVDCThyristorBased/Rectifier Control and Protection/Rectifier Protections/Low  AC Voltage Detection (LACVD) ==
  note: Low AC Voltage Detection
  Uac (pu) : Inport
  Enable (Held) : EnablePort  PropagateVarSize=During execution  ShowOutputPort=on
  C : Constant  Value=STATE
  LACVD : Subsystem  TreatAsAtomicUnit=on
  Logical Operator : Logic  AllPortsSameDT=off
  Low_AC_Voltage : Outport  VectorParamsAs1DForOutWhenUnconnected=off
  wires:
  Uac (pu)/1 -> LACVD/1(Uac (pu))
  LACVD/1(Low_AC_Voltage) -> Low_AC_Voltage/1
  Enable (Held)/1 -> Logical Operator/1
  Logical Operator/1 -> LACVD/Enable
  C/1 -> Logical Operator/2

== system HVDCThyristorBased/Rectifier Control and Protection/Rectifier Protections/Udio_6p ==
  note: Three-phase full-wave rectification
  Uabc (pu) : Inport
  MinMax : MinMax  Function=max  InputSameDT=on  SaturateOnIntegerOverflow=on
  MinMax1 : MinMax  InputSameDT=on  SaturateOnIntegerOverflow=on
  Sum : Sum  Inputs=+-  InputSameDT=on  SaturateOnIntegerOverflow=on  OutDataTypeStr=Inherit: Same as first input
  conversion pu ac->dc : Gain  Gain=pi/(3*sqrt(3))  SaturateOnIntegerOverflow=on  OutDataTypeStr=Inherit: Same as input  ParamDataTypeStr=Inherit: Same as input
  Udio_6p : Outport  VectorParamsAs1DForOutWhenUnconnected=off
  wires:
  conversion pu ac->dc/1 -> Udio_6p/1
  Sum/1 -> conversion pu ac->dc/1
  Uabc (pu)/1 -> MinMax1/1, MinMax/1
  MinMax/1 -> Sum/1
  MinMax1/1 -> Sum/2

== system HVDCThyristorBased/Inverter Control and Protection/Gamma Measurement/Gamma Measurement (D1 bridge)/Commutation Voltages ==
  note: Secondary Winding Connection
      | transfo_type : 1=Y  2=D1(lag)  3=D11(lead)
  note: Suppress
      |  zero- sequence voltages
  Uabc : Inport
  Constant3 : Constant  Value=transfo_type
  Gain1 : Gain  Gain=1/3  SaturateOnIntegerOverflow=on  OutDataTypeStr=Inherit: Same as input  ParamDataTypeStr=Inherit: Same as input
  Gain2 : Gain  Gain=sqrt(3)  SaturateOnIntegerOverflow=on  OutDataTypeStr=Inherit: Same as input  ParamDataTypeStr=Inherit: Same as input
  Gain3 : Gain  Gain=sqrt(3)  SaturateOnIntegerOverflow=on  OutDataTypeStr=Inherit: Same as input  ParamDataTypeStr=Inherit: Same as input
  Gain5 : Gain  Gain=-1  SaturateOnIntegerOverflow=on  OutDataTypeStr=Inherit: Same as input  ParamDataTypeStr=Inherit: Same as input
  Gain6 : Gain  Gain=-1  SaturateOnIntegerOverflow=on  OutDataTypeStr=Inherit: Same as input  ParamDataTypeStr=Inherit: Same as input
  Multiport Switch : MultiPortSwitch  InputSameDT=off
  Mux1 : Mux  Inputs=[3 3]
  Selector : Selector  InputPortWidth=3  IndexOptions=Index vector (dialog)  Indices=[2 3 1]  OutputSizes=1
  Selector1 : Selector  InputPortWidth=3  IndexOptions=Index vector (dialog)  Indices=[3 1 2]  OutputSizes=1
  Selector2 : Selector  InputPortWidth=6  IndexOptions=Index vector (dialog)  Indices="[1 4  2  5  3  6]"  OutputSizes=1
  Sum2 : Sum  Inputs=1  SaturateOnIntegerOverflow=on
  Sum3 : Sum  Inputs=|+-  SaturateOnIntegerOverflow=on
  Sum5 : Sum  Inputs=|++  SaturateOnIntegerOverflow=on
  Ucom (1-6) : Outport  VectorParamsAs1DForOutWhenUnconnected=off
  wires:
  Selector/1 -> Sum5/2, Gain3/1  "-Ub -Uc -Ua"
  Gain6/1 -> Selector/1
  Gain5/1 -> Selector1/1
  Constant3/1 -> Multiport Switch/1
  Sum5/1 -> Multiport Switch/2  "Uab Ubc Uca"
  Multiport Switch/1 -> Gain5/1, Mux1/1  "Ucom 1-3-5"
  Selector1/1 -> Mux1/2  "Ucom 2-4-6"
  Mux1/1 -> Selector2/1
  Uabc/1 -> Sum3/1, Sum2/1  "Uag Ubg Ucg"
  Sum2/1 -> Gain1/1
  Gain1/1 -> Sum3/2
  Sum3/1 -> Sum5/1, Gain2/1, Gain6/1  "Ua Ub Uc"
  Selector2/1 -> Ucom (1-6)/1
  Gain2/1 -> Multiport Switch/3
  Gain3/1 -> Multiport Switch/4

== system HVDCThyristorBased/Inverter Control and Protection/Gamma Measurement/Gamma Measurement (D1 bridge)/Pulse_counter_sampler (1-6) ==
  angles(1-6) : Inport
  Trigger : TriggerPort  VariantControl=Variant
  Add : Sum
  Constant : Constant  Value=6
  Constant1 : Constant
  Demux : Demux  Outputs=6
  Fcn : Fcn  Expr=(u[1]+1)
  Math Function : Math  Operator=mod  SignedPower=on
  Multiport Switch : MultiPortSwitch  Inputs=6  SaturateOnIntegerOverflow=off  InputSameDT=off
  Unit Delay : UnitDelay  SampleTime=-1  HasFrameUpgradeWarning=on
  angle : Outport  VectorParamsAs1DForOutWhenUnconnected=off
  pulse_n : Outport  Port=2  VectorParamsAs1DForOutWhenUnconnected=off
  wires:
  Demux/6 -> Multiport Switch/7
  Demux/5 -> Multiport Switch/6
  Demux/4 -> Multiport Switch/5
  Demux/3 -> Multiport Switch/4
  Demux/2 -> Multiport Switch/3
  Demux/1 -> Multiport Switch/2
  Fcn/1 -> Unit Delay/1, Math Function/1
  Unit Delay/1 -> Fcn/1
  Constant/1 -> Math Function/2
  Math Function/1 -> Add/2
  Constant1/1 -> Add/1
  Add/1 -> pulse_n/1, Multiport Switch/1
  Multiport Switch/1 -> angle/1
  angles(1-6)/1 -> Demux/1

== system HVDCThyristorBased/Inverter Control and Protection/Gamma Measurement/Gamma Measurement (D1 bridge)/Zero crossing interpolation ==
  note: Crossing time error evaluation (t_err) by linear interpolation
      | in a discrete system (sampling time is Ts)
  note: yb
  y : Inport
  Sample : Inport  Port=2
  Enable (Held) : EnablePort  PropagateVarSize=During execution
  (TOL) : simulink/Logic and Bit Operations/Compare To Constant  relop=>=  const=TOL  OutDataTypeStr=boolean  ZeroCross=off
  Abs : Abs
  Constant1 : Constant  Value=y0
  Constant4 : Constant  Value=inf
  Divide : Product  Inputs=*/
  Gain : Gain  Gain=Ts  SaturateOnIntegerOverflow=on  OutDataTypeStr=Inherit: Same as input  ParamDataTypeStr=Inherit: Same as input
  Min+0 Max=Ts : Saturate  UpperLimit=Ts  LowerLimit=0  SampleTime=Ts
  Sample and Hold : spsSampleandHoldLib/Sample and Hold  ic=0  Ts=Ts
  Subtract1 : Sum  Inputs=-+
  Subtract3 : Sum  Inputs=+-
  Switch : Switch  Criteria=u2 > Threshold  OutDataTypeStr=single  SampleTime=Ts
  Unit Delay : UnitDelay  SampleTime=Ts  HasFrameUpgradeWarning=on
  t_err : Outport  VectorParamsAs1DForOutWhenUnconnected=off
  wires:
  Gain/1 -> Divide/1
  Unit Delay/1 -> Subtract3/2  "ya"
  Subtract3/1 -> Abs/1, Switch/1
  Abs/1 -> (TOL)/1
  (TOL)/1 -> Switch/2
  Constant4/1 -> Switch/3
  Switch/1 -> Divide/2
  y/1 -> Unit Delay/1, Subtract3/1, Subtract1/2
  Divide/1 -> Min+0 Max=Ts/1  "correction"
  Constant1/1 -> Subtract1/1
  Subtract1/1 -> Gain/1
  Min+0 Max=Ts/1 -> Sample and Hold/1
  Sample and Hold/1 -> t_err/1
  Sample/1 -> Sample and Hold/2

== system HVDCThyristorBased/Inverter Control and Protection/Gamma Measurement/Gamma Measurement (Y bridge)/Commutation Voltages ==
  note: Secondary Winding Connection
      | transfo_type : 1=Y  2=D1(lag)  3=D11(lead)
  note: Suppress
      |  zero- sequence voltages
  Uabc : Inport
  Constant3 : Constant  Value=transfo_type
  Gain1 : Gain  Gain=1/3  SaturateOnIntegerOverflow=on  OutDataTypeStr=Inherit: Same as input  ParamDataTypeStr=Inherit: Same as input
  Gain2 : Gain  Gain=sqrt(3)  SaturateOnIntegerOverflow=on  OutDataTypeStr=Inherit: Same as input  ParamDataTypeStr=Inherit: Same as input
  Gain3 : Gain  Gain=sqrt(3)  SaturateOnIntegerOverflow=on  OutDataTypeStr=Inherit: Same as input  ParamDataTypeStr=Inherit: Same as input
  Gain5 : Gain  Gain=-1  SaturateOnIntegerOverflow=on  OutDataTypeStr=Inherit: Same as input  ParamDataTypeStr=Inherit: Same as input
  Gain6 : Gain  Gain=-1  SaturateOnIntegerOverflow=on  OutDataTypeStr=Inherit: Same as input  ParamDataTypeStr=Inherit: Same as input
  Multiport Switch : MultiPortSwitch  InputSameDT=off
  Mux1 : Mux  Inputs=[3 3]
  Selector : Selector  InputPortWidth=3  IndexOptions=Index vector (dialog)  Indices=[2 3 1]  OutputSizes=1
  Selector1 : Selector  InputPortWidth=3  IndexOptions=Index vector (dialog)  Indices=[3 1 2]  OutputSizes=1
  Selector2 : Selector  InputPortWidth=6  IndexOptions=Index vector (dialog)  Indices="[1 4  2  5  3  6]"  OutputSizes=1
  Sum2 : Sum  Inputs=1  SaturateOnIntegerOverflow=on
  Sum3 : Sum  Inputs=|+-  SaturateOnIntegerOverflow=on
  Sum5 : Sum  Inputs=|++  SaturateOnIntegerOverflow=on
  Ucom (1-6) : Outport  VectorParamsAs1DForOutWhenUnconnected=off
  wires:
  Selector/1 -> Sum5/2, Gain3/1  "-Ub -Uc -Ua"
  Gain6/1 -> Selector/1
  Gain5/1 -> Selector1/1
  Constant3/1 -> Multiport Switch/1
  Sum5/1 -> Multiport Switch/2  "Uab Ubc Uca"
  Multiport Switch/1 -> Gain5/1, Mux1/1  "Ucom 1-3-5"
  Selector1/1 -> Mux1/2  "Ucom 2-4-6"
  Mux1/1 -> Selector2/1
  Uabc/1 -> Sum3/1, Sum2/1  "Uag Ubg Ucg"
  Sum2/1 -> Gain1/1
  Gain1/1 -> Sum3/2
  Sum3/1 -> Sum5/1, Gain2/1, Gain6/1  "Ua Ub Uc"
  Selector2/1 -> Ucom (1-6)/1
  Gain2/1 -> Multiport Switch/3
  Gain3/1 -> Multiport Switch/4
